simulink model "Scan2SetPointDist"  (R2015b)
settings: Solver=FixedStepAuto  StartTime=0.0  StopTime=inf  FixedStep=0.05  RelTol=1e-3
libraries: robotlib x5
settings Model: Creator=einar  LastModifiedBy=Einar Ueland
settings OptimizationCC: OptimizeModelRefInitCode=on  LifeSpan=Inf  MaxStackSize=64
settings HardwareCC: ProdBitPerPointer=32  ProdLargestAtomicFloat=None  ProdIntDivRoundTo=Undefined  ProdEndianess=Unspecified  ProdWordSize=32  ProdHWDeviceType=Generic->Unspecified (assume 32-bit Generic)
settings RTWCC: SystemTargetFile=ert.tlc  TemplateMakefile=ert_default_tmf  Description=Embedded Coder  Toolchain=Catkin  TargetLang=C++
settings CodeAppCC: IgnoreCustomStorageClasses=off
settings ERTTargetCC: SupportContinuousTime=on  SupportVariableSizeSignals=on

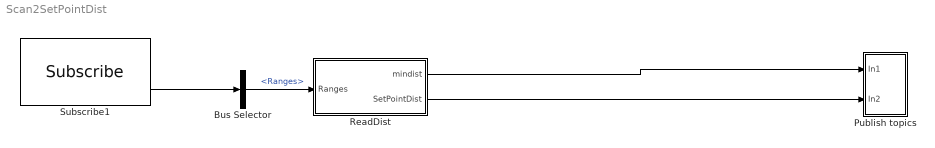
== system Scan2SetPointDist ==
  Bus Selector : BusSelector  OutputSignals=Ranges
  Publish topics : Subsystem
  ReadDist : MATLAB Function  TreatAsAtomicUnit=on
  Subscribe1 : robotlib/Subscribe  SourceLibraryInfo=This block requires Robotics System Toolbox  topicSource=Select from ROS network  topic=/scan  messageType=sensor_msgs/LaserScan  sampleTime=-1  messageQueueLength=1
  wires:
  Subscribe1/2 -> Bus Selector/1
  Bus Selector/1 -> ReadDist/1(Ranges)  "<Ranges>"
  ReadDist/1(mindist) -> Publish topics/1(In1)
  ReadDist/2(SetPointDist) -> Publish topics/2(In2)

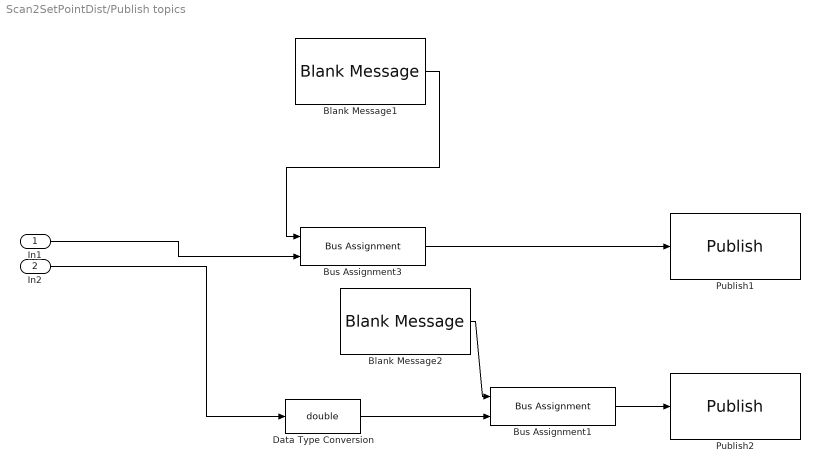
== system Scan2SetPointDist/Publish topics ==
  In1 : Inport
  In2 : Inport  Port=2
  Blank Message1 : robotlib/Blank Message  SourceLibraryInfo=This block requires Robotics System Toolbox  messageType=std_msgs/Float32  SampleTime=inf
  Blank Message2 : robotlib/Blank Message  SourceLibraryInfo=This block requires Robotics System Toolbox  messageType=std_msgs/Float64  SampleTime=inf
  Bus Assignment1 : BusAssignment  AssignedSignals=Data
  Bus Assignment3 : BusAssignment  AssignedSignals=Data
  Data Type Conversion : DataTypeConversion  OutDataTypeStr=double
  Publish1 : robotlib/Publish  SourceLibraryInfo=This block requires Robotics System Toolbox  topicSource=Specify your own  topic=/ScanDistance  messageType=std_msgs/Float32  messageQueueLength=1
  Publish2 : robotlib/Publish  SourceLibraryInfo=This block requires Robotics System Toolbox  topicSource=Specify your own  topic=/SetPointDist  messageType=std_msgs/Float64  messageQueueLength=1
  wires:
  Bus Assignment3/1 -> Publish1/1
  Blank Message1/1 -> Bus Assignment3/1
  Bus Assignment1/1 -> Publish2/1
  In1/1 -> Bus Assignment3/2
  Blank Message2/1 -> Bus Assignment1/1
  In2/1 -> Data Type Conversion/1
  Data Type Conversion/1 -> Bus Assignment1/2

== matlab function Scan2SetPointDist/ReadDist ==
  data: Ranges input; mindist output; SetPointDist output
function [mindist,SetPointDist] = fcn(Ranges)
%Find setpoint distance and minimal distance from lidar scann
mindist=min(Ranges);
if mindist<1
    SetPointDist=mindist-0.2;
else 
SetPointDist=2*mindist-1.2;
end
SetPointDist=min([SetPointDist 3])
SetPointDist=max([SetPointDist 0.1]);
end
